simulink model "QiMotorController_ModelReference"  (R2021b)
settings: Solver=FixedStepDiscrete  StartTime=0.0  StopTime=5  RelTol=1e-3
PreLoadFcn:
  | RTWConfigurationCB('preloadfcn', bdroot);
PostLoadFcn:
  | load('configuration/data_struct.mat');
  | load('configuration/fluxMaps_propMotor.mat');
  | load('configuration/parameterInit_PROP.mat');
  | load('configuration/parameterInit_PUMP.mat');
  | load('configuration/parameterInit_PITCH.mat');
  | load('configuration/parameterInit_TILT.mat');
  | %load('configuration/base_workspace_signal_definition.mat');
  | %load('resolvedatastores_to_baseworkspace_for_faster_simulation.mat');
model workspace (MAT data in the model file):
  ADC_CALIBRATION_SAMPLES : Simulink.Parameter (value not decoded)
  DEFAULT_RESOLVER_CONTROL_WORD : Simulink.Parameter (value not decoded)
  PLL_FREQUENCY : Simulink.Parameter (value not decoded)
  SIMULATION_OPTIONS : Simulink.Parameter (value not decoded)
  TARGET_CODE_GEN : Simulink.Parameter (value not decoded)
  Ts = 2.5e-07
symbols that are objects in the model workspace (value not decoded): PLL_FREQUENCY, TARGET_CODE_GEN
undefined symbols (not defined in the file): DEADTIME_NS__PITCH, DEADTIME_NS__PROP, DEADTIME_NS__PUMP, DEADTIME_NS__TILT, fIa_, fIb_, fIc_, fIdc_, fMotorEncoderFloat_, fMotorSensorSpeed_, fUa_, fUb_, fUc_, fUdc_, inbtilt, mdl_pitch_uiAPUFlags, mdl_pitch_uiFlags, modelData, oMot_, oOut_, opInputResolverData_, oPitch, oState_, PLANT_SPEED_QUADRATIC_COEFF__PUMP, POLE_PAIRS_INIT__PITCH, POLE_PAIRS_INIT__PROP, POLE_PAIRS_INIT__PUMP, POLE_PAIRS_INIT__TILT, PWM_FREQ_KHZ__PITCH, PWM_FREQ_KHZ__PROP, PWM_FREQ_KHZ__PUMP, R_PHASE_INIT__PITCH, R_PHASE_INIT__PROP, R_PHASE_INIT__TILT, R_PHASE_INIT_PLANT__PUMP, uiControlReadback_, uiGateDriverStatus_
libraries: simulink x51, spsSeriesRLCBranchLib x25, spsMosfetLib x24, powerlib_extras x24, spsCurrentMeasurementLib x17, spsVoltageMeasurementLib x17, spsPermanentMagnetSynchronousMachineLib x3, spsDCVoltageSourceLib x2, motorModelLibrary x2, slpidlib x2, cstblocks x1, spspowerguiLib x1
(part 3 of 5)

== system QiMotorController_ModelReference/pitchMotor/PWM_pitch ==
  pitchMotor_PWMticks : Inport
  Bus Creator1 : BusCreator  Inputs=6
  Center-Aligned PWM 3-Phase   Modulator2 : Subsystem
  Demux3 : Demux  Outputs=6
  Demux4 : Demux  Outputs=3
  Logical Operator{7..12} (6 alike) : Logic  IconShape=distinctive  AllPortsSameDT=off  OutDataTypeStr=boolean
  On Delay{6..11} (6 alike) : powerlib_extras/Discrete  Control Blocks/Discrete On//Off Delay  type_delay=On delay  delay=DEADTIME_NS__PITCH*10^-9  ic=0  Ts=Ts
      settings: SourceProductBaseCode=PS
  pitchMotor_enable : Constant  OutDataTypeStr=boolean  SampleTime=-1
  pitchMotor_PWMgates : Outport
  wires:
  Demux3/4 -> Logical Operator11/1
  Demux3/2 -> Logical Operator9/1
  Demux3/5 -> Logical Operator7/1
  pitchMotor_PWMticks/1 -> Demux4/1
  Logical Operator12/1 -> On Delay11/1
  Logical Operator8/1 -> On Delay6/1
  Demux4/3 -> Center-Aligned PWM 3-Phase   Modulator2/3(C_ticks)
  pitchMotor_enable/1 -> Logical Operator12/2, Logical Operator7/2, Logical Operator11/2, Logical Operator10/2, Logical Operator9/2, Logical Operator8/2
  Center-Aligned PWM 3-Phase   Modulator2/1(PWM Gates) -> Demux3/1
  Logical Operator9/1 -> On Delay7/1
  On Delay9/1 -> Bus Creator1/4  "pitchGate_Bbottom"
  Demux4/2 -> Center-Aligned PWM 3-Phase   Modulator2/2(B_ticks)
  Logical Operator7/1 -> On Delay10/1
  Demux3/6 -> Logical Operator12/1
  Demux4/1 -> Center-Aligned PWM 3-Phase   Modulator2/1(A_ticks)
  Demux3/3 -> Logical Operator10/1
  On Delay8/1 -> Bus Creator1/3  "pitchGate_Btop"
  On Delay11/1 -> Bus Creator1/6  "pitchGate_Cbottom"
  On Delay7/1 -> Bus Creator1/2  "pitchGate_Abottom"
  On Delay6/1 -> Bus Creator1/1  "pitchGate_Atop"
  On Delay10/1 -> Bus Creator1/5  "pitchGate_Ctop"
  Logical Operator11/1 -> On Delay9/1
  Bus Creator1/1 -> pitchMotor_PWMgates/1
  Demux3/1 -> Logical Operator8/1
  Logical Operator10/1 -> On Delay8/1

== system QiMotorController_ModelReference/pitchMotor/Sense1 ==
  Current Measurement : spsCurrentMeasurementLib/Current Measurement  Tag=PoWeRsYsTeMmEaSuReMeNt  PhasorSimulation=off  OutputType=Complex  PSBequivalent=0
      settings: AttributesFormatString=\n
  Current Measurement1 : spsCurrentMeasurementLib/Current Measurement  Tag=PoWeRsYsTeMmEaSuReMeNt  PhasorSimulation=off  OutputType=Complex  PSBequivalent=0
      settings: AttributesFormatString=\n
  Current Measurement2 : spsCurrentMeasurementLib/Current Measurement  Tag=PoWeRsYsTeMmEaSuReMeNt  PhasorSimulation=off  OutputType=Complex  PSBequivalent=0
      settings: AttributesFormatString=\n
  Mux1 : Mux  Inputs=3
  Mux2 : Mux  Inputs=3
  Rate Transition : RateTransition  OutPortSampleTime=Ts
  Rate Transition1 : RateTransition  OutPortSampleTime=Ts
  Voltage Measurement : spsVoltageMeasurementLib/Voltage Measurement  PhasorSimulation=off  OutputType=Complex  PSBequivalent=0
  Voltage Measurement1 : spsVoltageMeasurementLib/Voltage Measurement  PhasorSimulation=off  OutputType=Complex  PSBequivalent=0
  Voltage Measurement2 : spsVoltageMeasurementLib/Voltage Measurement  PhasorSimulation=off  OutputType=Complex  PSBequivalent=0
  Ta : PMIOPort  Side=Left
  Tb : PMIOPort  Port=2  Side=Left
  Tc : PMIOPort  Port=3  Side=Left
  Mta : PMIOPort  Port=4  Side=Right
  Mtb : PMIOPort  Port=5  Side=Right
  Mtc : PMIOPort  Port=6  Side=Right
  Neutral : PMIOPort  Port=7  Side=Left
  I_abc : Outport  SampleTime=Ts
  V_abc : Outport  Port=2
  wires:
  Mux1/1 -> Rate Transition/1
  Current Measurement1/1 -> Mux1/2
  Current Measurement/1 -> Mux1/1
  Current Measurement2/1 -> Mux1/3
  Voltage Measurement/1 -> Mux2/1  "Van"
  Voltage Measurement1/1 -> Mux2/2  "Vbn"
  Voltage Measurement2/1 -> Mux2/3  "Vcn"
  Rate Transition/1 -> I_abc/1
  Mux2/1 -> Rate Transition1/1
  Rate Transition1/1 -> V_abc/1
  connections:
  Current Measurement2/RConn1 -- Mtc/RConn1
  Tc/RConn1 -- Voltage Measurement2/LConn1 -- Current Measurement2/LConn1
  Ta/RConn1 -- Voltage Measurement/LConn1 -- Current Measurement/LConn1
  Current Measurement/RConn1 -- Mta/RConn1
  Tb/RConn1 -- Voltage Measurement1/LConn1 -- Current Measurement1/LConn1
  Current Measurement1/RConn1 -- Mtb/RConn1
  Neutral/RConn1 -- Voltage Measurement1/LConn2 -- Voltage Measurement2/LConn2 -- Voltage Measurement/LConn2

== system QiMotorController_ModelReference/propMotor/PWM_prop ==
  propMotor_PWMticks : Inport
  Bus Creator : BusCreator  Inputs=6
  Center-Aligned PWM 3-Phase   Modulator1 : Subsystem
  Demux1 : Demux  Outputs=3
  Demux2 : Demux  Outputs=6
  Logical Operator{1..6} (6 alike) : Logic  IconShape=distinctive  AllPortsSameDT=off  OutDataTypeStr=boolean
  On Delay{,1..5} (6 alike) : powerlib_extras/Discrete  Control Blocks/Discrete On//Off Delay  type_delay=On delay  delay=DEADTIME_NS__PROP*10^-9  ic=0  Ts=Ts
      settings: SourceProductBaseCode=PS
  propMotor_enable : Constant  OutDataTypeStr=boolean  SampleTime=-1
  propMotor_PWMgates : Outport
  wires:
  Demux2/5 -> Logical Operator1/1
  Demux1/1 -> Center-Aligned PWM 3-Phase   Modulator1/1(Ua)
  Demux2/3 -> Logical Operator4/1
  Logical Operator3/1 -> On Delay1/1
  Demux2/1 -> Logical Operator2/1
  On Delay3/1 -> Bus Creator/4  "propGate_Bbottom"
  Logical Operator6/1 -> On Delay5/1
  Demux2/2 -> Logical Operator3/1
  Bus Creator/1 -> propMotor_PWMgates/1
  On Delay2/1 -> Bus Creator/3  "propGate_Btop"
  Demux1/3 -> Center-Aligned PWM 3-Phase   Modulator1/3(Uc)
  On Delay1/1 -> Bus Creator/2  "propGate_Abottom"
  Center-Aligned PWM 3-Phase   Modulator1/1(PWM Gates) -> Demux2/1
  Demux2/4 -> Logical Operator5/1
  Logical Operator5/1 -> On Delay3/1
  propMotor_enable/1 -> Logical Operator6/2, Logical Operator1/2, Logical Operator5/2, Logical Operator4/2, Logical Operator3/2, Logical Operator2/2
  Demux1/2 -> Center-Aligned PWM 3-Phase   Modulator1/2(Ub)
  On Delay/1 -> Bus Creator/1  "propGate_Atop"
  On Delay5/1 -> Bus Creator/6  "propGate_Cbottom"
  Logical Operator4/1 -> On Delay2/1
  propMotor_PWMticks/1 -> Demux1/1
  Demux2/6 -> Logical Operator6/1
  On Delay4/1 -> Bus Creator/5  "propGate_Ctop"
  Logical Operator2/1 -> On Delay/1
  Logical Operator1/1 -> On Delay4/1

== system QiMotorController_ModelReference/propMotor/Sense1 ==
  Current Measurement : spsCurrentMeasurementLib/Current Measurement  Tag=PoWeRsYsTeMmEaSuReMeNt  PhasorSimulation=off  OutputType=Complex  PSBequivalent=0
      settings: AttributesFormatString=\n
  Current Measurement1 : spsCurrentMeasurementLib/Current Measurement  Tag=PoWeRsYsTeMmEaSuReMeNt  PhasorSimulation=off  OutputType=Complex  PSBequivalent=0
      settings: AttributesFormatString=\n
  Current Measurement2 : spsCurrentMeasurementLib/Current Measurement  Tag=PoWeRsYsTeMmEaSuReMeNt  PhasorSimulation=off  OutputType=Complex  PSBequivalent=0
      settings: AttributesFormatString=\n
  Mux1 : Mux  Inputs=3
  Mux2 : Mux  Inputs=3
  Rate Transition : RateTransition  OutPortSampleTime=Ts
  Rate Transition1 : RateTransition  OutPortSampleTime=Ts
  Voltage Measurement : spsVoltageMeasurementLib/Voltage Measurement  PhasorSimulation=off  OutputType=Complex  PSBequivalent=0
  Voltage Measurement1 : spsVoltageMeasurementLib/Voltage Measurement  PhasorSimulation=off  OutputType=Complex  PSBequivalent=0
  Voltage Measurement2 : spsVoltageMeasurementLib/Voltage Measurement  PhasorSimulation=off  OutputType=Complex  PSBequivalent=0
  Ta : PMIOPort  Side=Left
  Tb : PMIOPort  Port=2  Side=Left
  Tc : PMIOPort  Port=3  Side=Left
  Mta : PMIOPort  Port=4  Side=Right
  Mtb : PMIOPort  Port=5  Side=Right
  Mtc : PMIOPort  Port=6  Side=Right
  Neutral : PMIOPort  Port=7  Side=Left
  I_abc : Outport  SampleTime=Ts
  V_abc : Outport  Port=2
  wires:
  Mux1/1 -> Rate Transition/1
  Current Measurement1/1 -> Mux1/2
  Current Measurement/1 -> Mux1/1
  Current Measurement2/1 -> Mux1/3
  Voltage Measurement/1 -> Mux2/1  "Van"
  Voltage Measurement1/1 -> Mux2/2  "Vbn"
  Voltage Measurement2/1 -> Mux2/3  "Vcn"
  Rate Transition/1 -> I_abc/1
  Mux2/1 -> Rate Transition1/1
  Rate Transition1/1 -> V_abc/1
  connections:
  Current Measurement2/RConn1 -- Mtc/RConn1
  Tc/RConn1 -- Voltage Measurement2/LConn1 -- Current Measurement2/LConn1
  Ta/RConn1 -- Voltage Measurement/LConn1 -- Current Measurement/LConn1
  Current Measurement/RConn1 -- Mta/RConn1
  Tb/RConn1 -- Voltage Measurement1/LConn1 -- Current Measurement1/LConn1
  Current Measurement1/RConn1 -- Mtb/RConn1
  Neutral/RConn1 -- Voltage Measurement1/LConn2 -- Voltage Measurement2/LConn2 -- Voltage Measurement/LConn2

== system QiMotorController_ModelReference/propMotor/Sim Option Prop Variant Subsystem ==
  note: 1) Add Subsystem or Model blocks as valid variant choices.
      | 2) You cannot connect blocks at this level. At simulation, connectivity is automatically
      | determined, based on the active variant and port name matching.
  In1 : Inport
  Sim Options 0 Prop Subsystem : Subsystem  VariantControl=(default)
  Sim Options 1 Prop Subsystem : Subsystem  VariantControl=SIMULATION_OPTIONS == 1 && TARGET_CODE_GEN ~= 1
  Out1 : Outport

== system QiMotorController_ModelReference/pumpfanMotor/PWM_pumpfan ==
  pumpMotor_PWMticks : Inport
  Bus Creator : BusCreator  Inputs=6
  Center-Aligned PWM 3-Phase   Modulator1 : Subsystem
  Demux1 : Demux  Outputs=3
  Demux2 : Demux  Outputs=6
  Logical Operator{1..6} (6 alike) : Logic  IconShape=distinctive  AllPortsSameDT=off  OutDataTypeStr=boolean
  On Delay{,1..5} (6 alike) : powerlib_extras/Discrete  Control Blocks/Discrete On//Off Delay  type_delay=On delay  delay=DEADTIME_NS__PUMP*10^-9  ic=0  Ts=Ts
      settings: SourceProductBaseCode=PS
  pumpMotor_enable : Constant  OutDataTypeStr=boolean  SampleTime=-1
  pumpMotor_PWMgates : Outport
  wires:
  Demux2/5 -> Logical Operator1/1
  Demux1/1 -> Center-Aligned PWM 3-Phase   Modulator1/1(Ua)
  Demux2/3 -> Logical Operator4/1
  Logical Operator3/1 -> On Delay1/1
  Demux2/1 -> Logical Operator2/1
  On Delay3/1 -> Bus Creator/4  "pumpGate_Bbottom"
  Logical Operator6/1 -> On Delay5/1
  Demux2/2 -> Logical Operator3/1
  Bus Creator/1 -> pumpMotor_PWMgates/1
  On Delay2/1 -> Bus Creator/3  "pumpGate_Btop"
  Demux1/3 -> Center-Aligned PWM 3-Phase   Modulator1/3(Uc)
  On Delay1/1 -> Bus Creator/2  "pumpGate_Abottom"
  Center-Aligned PWM 3-Phase   Modulator1/1(PWM Gates) -> Demux2/1
  Demux2/4 -> Logical Operator5/1
  Logical Operator5/1 -> On Delay3/1
  pumpMotor_enable/1 -> Logical Operator6/2, Logical Operator1/2, Logical Operator5/2, Logical Operator4/2, Logical Operator3/2, Logical Operator2/2
  Demux1/2 -> Center-Aligned PWM 3-Phase   Modulator1/2(Ub)
  On Delay/1 -> Bus Creator/1  "pumpGate_Atop"
  On Delay5/1 -> Bus Creator/6  "pumpGate_Cbottom"
  Logical Operator4/1 -> On Delay2/1
  pumpMotor_PWMticks/1 -> Demux1/1
  Demux2/6 -> Logical Operator6/1
  On Delay4/1 -> Bus Creator/5  "pumpGate_Ctop"
  Logical Operator2/1 -> On Delay/1
  Logical Operator1/1 -> On Delay4/1

== system QiMotorController_ModelReference/pumpfanMotor/Sense1 ==
  Current Measurement : spsCurrentMeasurementLib/Current Measurement  Tag=PoWeRsYsTeMmEaSuReMeNt  PhasorSimulation=off  OutputType=Complex  PSBequivalent=0
      settings: AttributesFormatString=\n
  Current Measurement1 : spsCurrentMeasurementLib/Current Measurement  Tag=PoWeRsYsTeMmEaSuReMeNt  PhasorSimulation=off  OutputType=Complex  PSBequivalent=0
      settings: AttributesFormatString=\n
  Current Measurement2 : spsCurrentMeasurementLib/Current Measurement  Tag=PoWeRsYsTeMmEaSuReMeNt  PhasorSimulation=off  OutputType=Complex  PSBequivalent=0
      settings: AttributesFormatString=\n
  Mux1 : Mux  Inputs=3
  Mux2 : Mux  Inputs=3
  Rate Transition : RateTransition  OutPortSampleTime=Ts
  Rate Transition1 : RateTransition  OutPortSampleTime=Ts
  Voltage Measurement : spsVoltageMeasurementLib/Voltage Measurement  PhasorSimulation=off  OutputType=Complex  PSBequivalent=0
  Voltage Measurement1 : spsVoltageMeasurementLib/Voltage Measurement  PhasorSimulation=off  OutputType=Complex  PSBequivalent=0
  Voltage Measurement2 : spsVoltageMeasurementLib/Voltage Measurement  PhasorSimulation=off  OutputType=Complex  PSBequivalent=0
  Ta : PMIOPort  Side=Left
  Tb : PMIOPort  Port=2  Side=Left
  Tc : PMIOPort  Port=3  Side=Left
  Mta : PMIOPort  Port=4  Side=Right
  Mtb : PMIOPort  Port=5  Side=Right
  Mtc : PMIOPort  Port=6  Side=Right
  Neutral : PMIOPort  Port=7  Side=Left
  I_abc : Outport  SampleTime=Ts
  V_abc : Outport  Port=2
  wires:
  Mux1/1 -> Rate Transition/1
  Current Measurement1/1 -> Mux1/2
  Current Measurement/1 -> Mux1/1
  Current Measurement2/1 -> Mux1/3
  Voltage Measurement/1 -> Mux2/1  "Van"
  Voltage Measurement1/1 -> Mux2/2  "Vbn"
  Voltage Measurement2/1 -> Mux2/3  "Vcn"
  Rate Transition/1 -> I_abc/1
  Mux2/1 -> Rate Transition1/1
  Rate Transition1/1 -> V_abc/1
  connections:
  Current Measurement2/RConn1 -- Mtc/RConn1
  Tc/RConn1 -- Voltage Measurement2/LConn1 -- Current Measurement2/LConn1
  Ta/RConn1 -- Voltage Measurement/LConn1 -- Current Measurement/LConn1
  Current Measurement/RConn1 -- Mta/RConn1
  Tb/RConn1 -- Voltage Measurement1/LConn1 -- Current Measurement1/LConn1
  Current Measurement1/RConn1 -- Mtb/RConn1
  Neutral/RConn1 -- Voltage Measurement1/LConn2 -- Voltage Measurement2/LConn2 -- Voltage Measurement/LConn2

== system QiMotorController_ModelReference/pumpfanMotor/Sim Option Pump Variant Subsystem ==
  note: 1) Add Subsystem or Model blocks as valid variant choices.
      | 2) You cannot connect blocks at this level. At simulation, connectivity is automatically
      | determined, based on the active variant and port name matching.
  In1 : Inport
  Sim Options 0 Pump Subsystem : Subsystem  VariantControl=(default)
  Sim Options 1 Pump Subsystem : Subsystem  VariantControl=SIMULATION_OPTIONS == 1 && TARGET_CODE_GEN ~= 1
  Out1 : Outport

== system QiMotorController_ModelReference/tiltMotor/PWM_tilt ==
  tiltMotor_PWMticks : Inport
  Bus Creator1 : BusCreator  Inputs=6
  Center-Aligned PWM 3-Phase   Modulator2 : Subsystem
  Demux3 : Demux  Outputs=6
  Demux4 : Demux  Outputs=3
  Logical Operator{7..12} (6 alike) : Logic  IconShape=distinctive  AllPortsSameDT=off  OutDataTypeStr=boolean
  On Delay{6..11} (6 alike) : powerlib_extras/Discrete  Control Blocks/Discrete On//Off Delay  type_delay=On delay  delay=DEADTIME_NS__TILT*10^-9  ic=0  Ts=Ts
      settings: SourceProductBaseCode=PS
  tiltMotor_enable : Constant  OutDataTypeStr=boolean  SampleTime=-1
  tiltMotor_PWMgates : Outport
  wires:
  Demux3/4 -> Logical Operator11/1
  Demux3/2 -> Logical Operator9/1
  Demux3/5 -> Logical Operator7/1
  tiltMotor_PWMticks/1 -> Demux4/1
  Logical Operator12/1 -> On Delay11/1
  Logical Operator8/1 -> On Delay6/1
  Demux4/3 -> Center-Aligned PWM 3-Phase   Modulator2/3(C_ticks)
  tiltMotor_enable/1 -> Logical Operator12/2, Logical Operator7/2, Logical Operator11/2, Logical Operator10/2, Logical Operator9/2, Logical Operator8/2
  Center-Aligned PWM 3-Phase   Modulator2/1(PWM Gates) -> Demux3/1
  Logical Operator9/1 -> On Delay7/1
  On Delay9/1 -> Bus Creator1/4  "tiltGate_Bbottom"
  Demux4/2 -> Center-Aligned PWM 3-Phase   Modulator2/2(B_ticks)
  Logical Operator7/1 -> On Delay10/1
  Demux3/6 -> Logical Operator12/1
  Demux4/1 -> Center-Aligned PWM 3-Phase   Modulator2/1(A_ticks)
  Demux3/3 -> Logical Operator10/1
  On Delay8/1 -> Bus Creator1/3  "tiltGate_Btop"
  On Delay11/1 -> Bus Creator1/6  "tiltGate_Cbottom"
  On Delay7/1 -> Bus Creator1/2  "tiltGate_Abottom"
  On Delay6/1 -> Bus Creator1/1  "tiltGate_Atop"
  On Delay10/1 -> Bus Creator1/5  "tiltGate_Ctop"
  Logical Operator11/1 -> On Delay9/1
  Bus Creator1/1 -> tiltMotor_PWMgates/1
  Demux3/1 -> Logical Operator8/1
  Logical Operator10/1 -> On Delay8/1

== system QiMotorController_ModelReference/tiltMotor/Sense1 ==
  Current Measurement : spsCurrentMeasurementLib/Current Measurement  Tag=PoWeRsYsTeMmEaSuReMeNt  PhasorSimulation=off  OutputType=Complex  PSBequivalent=0
      settings: AttributesFormatString=\n
  Current Measurement1 : spsCurrentMeasurementLib/Current Measurement  Tag=PoWeRsYsTeMmEaSuReMeNt  PhasorSimulation=off  OutputType=Complex  PSBequivalent=0
      settings: AttributesFormatString=\n
  Current Measurement2 : spsCurrentMeasurementLib/Current Measurement  Tag=PoWeRsYsTeMmEaSuReMeNt  PhasorSimulation=off  OutputType=Complex  PSBequivalent=0
      settings: AttributesFormatString=\n
  Mux1 : Mux  Inputs=3
  Mux2 : Mux  Inputs=3
  Rate Transition : RateTransition  OutPortSampleTime=Ts
  Rate Transition1 : RateTransition  OutPortSampleTime=Ts
  Voltage Measurement : spsVoltageMeasurementLib/Voltage Measurement  PhasorSimulation=off  OutputType=Complex  PSBequivalent=0
  Voltage Measurement1 : spsVoltageMeasurementLib/Voltage Measurement  PhasorSimulation=off  OutputType=Complex  PSBequivalent=0
  Voltage Measurement2 : spsVoltageMeasurementLib/Voltage Measurement  PhasorSimulation=off  OutputType=Complex  PSBequivalent=0
  Ta : PMIOPort  Side=Left
  Tb : PMIOPort  Port=2  Side=Left
  Tc : PMIOPort  Port=3  Side=Left
  Mta : PMIOPort  Port=4  Side=Right
  Mtb : PMIOPort  Port=5  Side=Right
  Mtc : PMIOPort  Port=6  Side=Right
  Neutral : PMIOPort  Port=7  Side=Left
  I_abc : Outport  SampleTime=Ts
  V_abc : Outport  Port=2
  wires:
  Mux1/1 -> Rate Transition/1
  Current Measurement1/1 -> Mux1/2
  Current Measurement/1 -> Mux1/1
  Current Measurement2/1 -> Mux1/3
  Voltage Measurement/1 -> Mux2/1  "Van"
  Voltage Measurement1/1 -> Mux2/2  "Vbn"
  Voltage Measurement2/1 -> Mux2/3  "Vcn"
  Rate Transition/1 -> I_abc/1
  Mux2/1 -> Rate Transition1/1
  Rate Transition1/1 -> V_abc/1
  connections:
  Current Measurement2/RConn1 -- Mtc/RConn1
  Tc/RConn1 -- Voltage Measurement2/LConn1 -- Current Measurement2/LConn1
  Ta/RConn1 -- Voltage Measurement/LConn1 -- Current Measurement/LConn1
  Current Measurement/RConn1 -- Mta/RConn1
  Tb/RConn1 -- Voltage Measurement1/LConn1 -- Current Measurement1/LConn1
  Current Measurement1/RConn1 -- Mtb/RConn1
  Neutral/RConn1 -- Voltage Measurement1/LConn2 -- Voltage Measurement2/LConn2 -- Voltage Measurement/LConn2

== system QiMotorController_ModelReference/Fault Injection/pitchMotor_faults/DC Current Disturbance ==
  Idc_feedback : Inport
  Idc_value : Inport  Port=2
  Abs1 : Abs
  Constant2 : Constant  Value=0  OutDataTypeStr=single  SampleTime=-1
  GreaterThan1 : RelationalOperator  Operator=>  OutDataTypeStr=boolean  RndMeth=Simplest
  Switch : Switch  Criteria=u2 > Threshold
  Idc_fault : Outport
  wires:
  Idc_feedback/1 -> Switch/3
  GreaterThan1/1 -> Switch/2
  Switch/1 -> Idc_fault/1
  Idc_value/1 -> Switch/1, Abs1/1
  Constant2/1 -> GreaterThan1/2
  Abs1/1 -> GreaterThan1/1

== system QiMotorController_ModelReference/Fault Injection/pitchMotor_faults/DC Voltage Disturbance ==
  Udc_feedback : Inport
  Udc_value : Inport  Port=2
  Constant1 : Constant  Value=0  OutDataTypeStr=single  SampleTime=-1
  GreaterThan : RelationalOperator  Operator=>  OutDataTypeStr=boolean  RndMeth=Simplest
  Switch : Switch  Criteria=u2 > Threshold
  Udc_fault : Outport
  wires:
  Udc_value/1 -> Switch/1, GreaterThan/1
  GreaterThan/1 -> Switch/2
  Constant1/1 -> GreaterThan/2
  Udc_feedback/1 -> Switch/3
  Switch/1 -> Udc_fault/1

== system QiMotorController_ModelReference/Fault Injection/pitchMotor_faults/Phase Current & Aux Disturbances ==
  note: This simulates a HW overcurrent fault (1008) coming from the FPGA.
      | Takes precedence over other faults.
  Iabc_feedback : Inport
  IphMagnitude_value : Inport  Port=2
  Target_phase : Inport  Port=3
  Aux_trip_code : Inport  Port=4
  uiGateDriverStatus : Inport  Port=5
  mdl_pitch_uiFlags : Inport  Port=6
  mdl_pitch_uiAPUFlags : Inport  Port=7
  Constant : Constant  Value=0xF  OutDataTypeStr=uint32  SampleTime=-1
  Constant2 : Constant  Value=10  OutDataTypeStr=single  SampleTime=-1
  Fault Current Setting : Subsystem
  GreaterThan1 : RelationalOperator  Operator=>  OutDataTypeStr=boolean  RndMeth=Simplest
  Set uiAPUFlags for Aux Trips : Subsystem  TreatAsAtomicUnit=on
  Set uiFlags for Aux Trips : Subsystem  TreatAsAtomicUnit=on
  Set uiGateDriverStatus for Aux Trips : Subsystem  TreatAsAtomicUnit=on
  Switch1 : Switch  Criteria=u2 > Threshold
  Iabc_fault : Outport
  uiGateDriverStatus_fault : Outport  Port=2
  uiFlags_fault : Outport  Port=3
  uiAPUFlags_fault : Outport  Port=4
  wires:
  IphMagnitude_value/1 -> Fault Current Setting/3(IphMagnitude_value), GreaterThan1/1
  Constant2/1 -> GreaterThan1/2
  GreaterThan1/1 -> Switch1/2
  Switch1/1 -> uiGateDriverStatus_fault/1
  Constant/1 -> Switch1/1
  Target_phase/1 -> Fault Current Setting/1(targetPhase)
  Aux_trip_code/1 -> Set uiAPUFlags for Aux Trips/1(auxTripCode), Set uiFlags for Aux Trips/1(auxTripCode), Set uiGateDriverStatus for Aux Trips/1(auxTripCode)
  mdl_pitch_uiFlags/1 -> Set uiFlags for Aux Trips/2(uiFlags)
  uiGateDriverStatus/1 -> Set uiGateDriverStatus for Aux Trips/2(uiGateDriverStatus)
  Set uiGateDriverStatus for Aux Trips/1(uiGateDriverStatus_fault) -> Switch1/3
  Set uiFlags for Aux Trips/1(uiFlags_fault) -> uiFlags_fault/1
  Iabc_feedback/1 -> Fault Current Setting/2(Iabc_feedback)
  Fault Current Setting/1(Iabc_fault) -> Iabc_fault/1
  Set uiAPUFlags for Aux Trips/1(uiAPUFlags_fault) -> uiAPUFlags_fault/1
  mdl_pitch_uiAPUFlags/1 -> Set uiAPUFlags for Aux Trips/2(uiAPUFlags)

== system QiMotorController_ModelReference/Fault Injection/pitchMotor_faults/Position Control Disturbances ==
  uiControlFeedback : Inport
  uiControlFeedback_value : Inport  Port=2
  Constant1 : Constant  Value=0  OutDataTypeStr=uint32  SampleTime=-1
  Constant2 : Constant  Value=0  OutDataTypeStr=uint32  SampleTime=-1
  GreaterThan1 : RelationalOperator  Operator=>  OutDataTypeStr=boolean  RndMeth=Simplest
  Switch : Switch  Criteria=u2 > Threshold
  uiControlFeedback_fault : Outport
  wires:
  uiControlFeedback/1 -> Switch/3
  GreaterThan1/1 -> Switch/2
  Switch/1 -> uiControlFeedback_fault/1
  uiControlFeedback_value/1 -> GreaterThan1/1
  Constant2/1 -> GreaterThan1/2
  Constant1/1 -> Switch/1

== system QiMotorController_ModelReference/InboardTiltDragLaw2/drag2/coulomb_drag_logic ==
  Bus Element In2 : Inport  PortName=velocity_m
  Bus Element In : Inport  Port=2  PortName=net_torque_m
  Bus Element In3 : Inport  Port=2  PortName=net_torque_m
  Bus Element In1 : Inport  Port=3  PortName=nominal_drag_torque_m
  Bus Element In4 : Inport  Port=3  PortName=nominal_drag_torque_m
  AND : Logic  IconShape=distinctive  AllPortsSameDT=off  OutDataTypeStr=boolean
  Abs5 : Abs
  Equal : RelationalOperator  Operator=<  OutDataTypeStr=boolean  RndMeth=Simplest
  Less Than : RelationalOperator  Operator=<  OutDataTypeStr=boolean  RndMeth=Simplest
  Product1 : Product
  Sign1 : Signum
  Switch : Switch  Criteria=u2 > Threshold
  minimum_stick_slip_velocity : Constant  Value=2e-1  OutDataTypeStr=Inherit: Inherit via back propagation
  Bus Element Out : Outport  PortName=drag_torque_out_m
  wires:
  Product1/1 -> Bus Element Out/1  "drag"
  Switch/1 -> Product1/2
  Sign1/1 -> Product1/1  "sgn"
  Bus Element In4/1 -> Switch/3
  Bus Element In1/1 -> Less Than/2  "nomtq"
  Bus Element In3/1 -> Switch/1  "nettq"
  Less Than/1 -> AND/2
  AND/1 -> Switch/2  "drag_conditional"
  Bus Element In2/1 -> Abs5/1, Sign1/1  "vm"
  Abs5/1 -> Equal/1
  Equal/1 -> AND/1
  minimum_stick_slip_velocity/1 -> Equal/2
  Bus Element In/1 -> Less Than/1  "nettq"

== system QiMotorController_ModelReference/InboardTiltDragLaw2/drag2/load ==
  Bus Element In4 : Inport  PortName=velocity_m
  Bus Element In1 : Inport  Port=2  PortName=ideal_load_torque_m
  Bus Element In2 : Inport  Port=2  PortName=ideal_load_torque_m
  Bus Element In3 : Inport  Port=2  PortName=ideal_load_torque_m
  Bus Element In14 : Inport  Port=3  PortName=motor_temp
  Bus Element In5 : Inport  Port=4  PortName=n_invs
  Abs2 : Abs
  Display : Display
  Display1 : Display
  Product : Product
  Product2 : Product
  Switch : Switch  Criteria=u2 > Threshold
  direct_efficiency : Subsystem
  e1 : Lookup_n-D  BreakpointsForDimension1=inbtilt.EfficiencyTemperatureBreakpoints  BreakpointsForDimension2=inbtilt.EfficiencySpeedBreakpoints  Table=inbtilt.EfficiencyTable  InternalRulePriority=Speed  RndMeth=Simplest  InputSameDT=on
      settings: InputPortMap=u0,u1
  indirect_efficiency_reduction : Subsystem
  Bus Element Out1 : Outport  PortName=load_torque
  wires:
  e1/1 -> direct_efficiency/1(table_efficiency)
  Bus Element In3/1 -> direct_efficiency/3(ideal_load_torque_m)
  Bus Element In2/1 -> Product2/2, Display/1
  Product2/1 -> Bus Element Out1/1
  Bus Element In1/1 -> indirect_efficiency_reduction/1(torque_load_m)
  indirect_efficiency_reduction/1(efficiency_load_reduction) -> Product/2
  Product/1 -> Switch/3  "e_indirect"
  Bus Element In5/1 -> Switch/2
  Switch/1 -> Product2/1, Display1/1  "e"
  direct_efficiency/1(nominal_efficiency) -> Switch/1, Product/1  "e_direct"
  Abs2/1 -> e1/2  "vm"
  Bus Element In14/1 -> e1/1  "T"
  Bus Element In4/1 -> direct_efficiency/2(velocity_m), Abs2/1

== system QiMotorController_ModelReference/Signal Conditioning/qi_dsm_to_sinc1/compute_dsm_output ==
  sig_in : Inport
  Add : Sum  Inputs=+-
  Add{1,3..7} (6 alike) : Sum
  Add2 : Sum  Inputs=+-
  Compare To Constant : simulink/Logic and Bit Operations/Compare To Constant  relop=>=  const=0  OutDataTypeStr=boolean
  Constant : Constant  SampleTime=-1
  Constant1 : Constant  Value=0  SampleTime=-1
  Constant2 : Constant  SampleTime=-1
  Constant3 : Constant  Value=2  SampleTime=-1
  Divide{,1..7} (8 alike) : Product  Inputs=**
  Switch : Switch  Criteria=u2 > Threshold
  Switch1 : Switch  Criteria=u2 > Threshold
  Switch2 : Switch  Criteria=u2 > Threshold
  Unit Delay{,1..6} (7 alike) : UnitDelay  SampleTime=-1  HasFrameUpgradeWarning=on
  pdm_signal : Outport
  wires:
  [b2] -> Divide/1
  [vref] -> Divide/2
  [s1_accum] -> Unit Delay1/1
  Divide/1 -> Add/2
  [s2_accum] -> Unit Delay/1
  [a2] -> Divide1/1
  Add/1 -> Divide1/2
  Unit Delay1/1 -> Add/1
  Unit Delay/1 -> Add1/1
  Divide1/1 -> Add1/2
  [vref] -> Divide2/2
  [b1] -> Divide2/1
  Divide2/1 -> Add2/2
  [a1] -> Divide3/1
  Add2/1 -> Divide3/2
  [s1_accum] -> Unit Delay2/1
  Unit Delay2/1 -> Add3/1
  Divide3/1 -> Add3/2
  [s2_accum] -> Unit Delay3/1
  Unit Delay3/1 -> Compare To Constant/1
  Add1/1 -> Switch/1
  Add3/1 -> Switch1/1
  Switch1/1 -> [s1_accum]
  Switch/1 -> [s2_accum]
  Compare To Constant/1 -> Switch1/2, Switch/2, Switch2/2
  Switch2/1 -> [dout], pdm_signal/1
  Constant/1 -> Switch2/1
  Constant1/1 -> Switch2/3
  [s2_accum] -> Unit Delay4/1
  Unit Delay4/1 -> Add5/1
  [s1_accum] -> Unit Delay5/1
  [a2] -> Divide5/1
  [vref] -> Divide4/2
  Add4/1 -> Divide5/2
  Unit Delay5/1 -> Add4/1
  [b2] -> Divide4/1
  Add5/1 -> Switch/3
  Divide5/1 -> Add5/2
  Divide4/1 -> Add4/2
  [s1_accum] -> Unit Delay6/1
  [b1] -> Divide6/1
  Divide7/1 -> Add7/2
  Add7/1 -> Switch1/3
  [a1] -> Divide7/1
  sig_in/1 -> Add6/1, Add2/1
  Add6/1 -> Divide7/2
  Unit Delay6/1 -> Add7/1
  [vref] -> Divide6/2
  Divide6/1 -> Add6/2
  Constant2/1 -> [a2], [vref], [b1], [a1]
  Constant3/1 -> [b2]

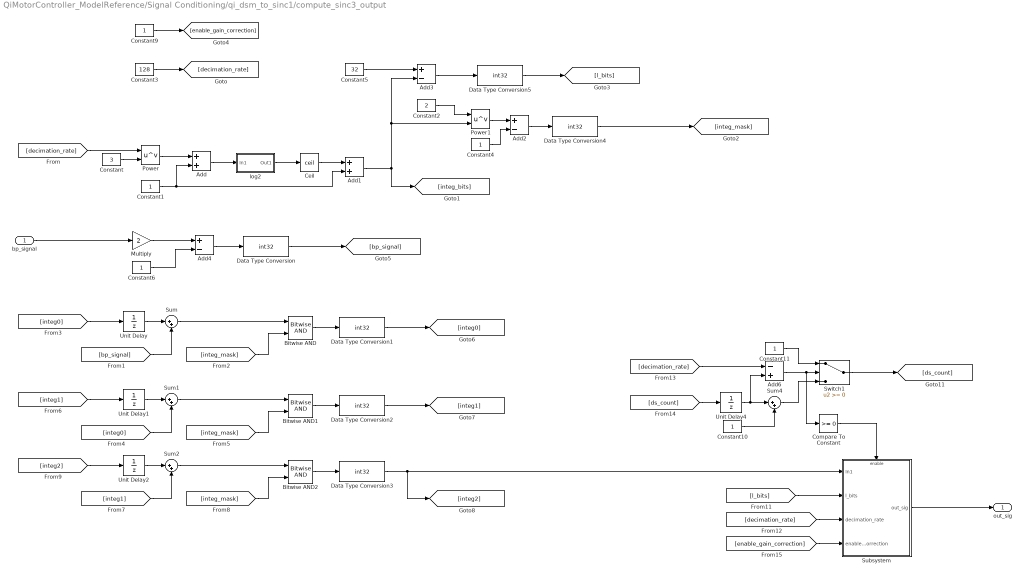
== system QiMotorController_ModelReference/Signal Conditioning/qi_dsm_to_sinc1/compute_sinc3_output ==
  bp_signal : Inport
  Add : Sum
  Add1 : Sum
  Add2 : Sum  Inputs=+-
  Add3 : Sum  Inputs=+-
  Add4 : Sum  Inputs=+-  OutDataTypeStr=int32
  Add6 : Sum  Inputs=-+  OutDataTypeStr=int32
  Bitwise AND : simulink/Logic and Bit Operations/Bitwise Operator  logicop=AND  UseBitMask=off  NumInputPorts=2  BitMask=bin2dec('11011001')  BitMaskRealWorld=Stored Integer
  Bitwise AND1 : simulink/Logic and Bit Operations/Bitwise Operator  logicop=AND  UseBitMask=off  NumInputPorts=2  BitMask=bin2dec('11011001')  BitMaskRealWorld=Stored Integer
  Bitwise AND2 : simulink/Logic and Bit Operations/Bitwise Operator  logicop=AND  UseBitMask=off  NumInputPorts=2  BitMask=bin2dec('11011001')  BitMaskRealWorld=Stored Integer
  Ceil : Rounding  Operator=ceil
  Compare To Constant : simulink/Logic and Bit Operations/Compare To Constant  relop=>=  const=0  OutDataTypeStr=boolean
  Constant : Constant  Value=3  OutDataTypeStr=single  SampleTime=-1
  Constant1 : Constant  OutDataTypeStr=single  SampleTime=-1
  Constant10 : Constant  OutDataTypeStr=int32  SampleTime=-1
  Constant11 : Constant  OutDataTypeStr=int32  SampleTime=-1
  Constant2 : Constant  Value=2  OutDataTypeStr=single  SampleTime=-1
  Constant3 : Constant  Value=128  OutDataTypeStr=single  SampleTime=-1
  Constant4 : Constant  OutDataTypeStr=single  SampleTime=-1
  Constant5 : Constant  Value=32  OutDataTypeStr=single  SampleTime=-1
  Constant6 : Constant  OutDataTypeStr=single  SampleTime=-1
  Constant9 : Constant  OutDataTypeStr=boolean  SampleTime=-1
  Data Type Conversion{,1..5} (6 alike) : DataTypeConversion  OutDataTypeStr=int32
  Multiply : Gain  Gain=2
  Power : Math  Operator=pow  SaturateOnIntegerOverflow=on
  Power1 : Math  Operator=pow  SaturateOnIntegerOverflow=on
  Subsystem : Subsystem
  Sum{,1..2,4} (4 alike) : Sum  Inputs=|++
  Switch1 : Switch
  Unit Delay : UnitDelay  SampleTime=-1  HasFrameUpgradeWarning=on
  Unit Delay1 : UnitDelay  SampleTime=-1  HasFrameUpgradeWarning=on
  Unit Delay2 : UnitDelay  SampleTime=-1  HasFrameUpgradeWarning=on
  Unit Delay4 : UnitDelay  InitialCondition=1  SampleTime=-1  HasFrameUpgradeWarning=on
  log2 : Subsystem
  out_sig : Outport
  wires:
  [decimation_rate] -> Power/1
  Constant/1 -> Power/2
  Power/1 -> Add/1
  Constant1/1 -> Add1/2, Add/2
  Constant3/1 -> [decimation_rate]
  Add/1 -> log2/1(In1)
  log2/1(Out1) -> Ceil/1
  Ceil/1 -> Add1/1
  Add1/1 -> Add3/2, Power1/2, [integ_bits]
  Constant2/1 -> Power1/1
  Power1/1 -> Add2/1
  Constant4/1 -> Add2/2
  Add2/1 -> Data Type Conversion4/1
  Constant5/1 -> Add3/1
  Add3/1 -> Data Type Conversion5/1
  bp_signal/1 -> Multiply/1
  Multiply/1 -> Add4/1
  Constant6/1 -> Add4/2
  Add4/1 -> Data Type Conversion/1
  Data Type Conversion/1 -> [bp_signal]
  Sum/1 -> Bitwise AND/1
  Unit Delay/1 -> Sum/1
  [bp_signal] -> Sum/2
  [integ_mask] -> Bitwise AND/2
  Bitwise AND/1 -> Data Type Conversion1/1
  Data Type Conversion1/1 -> [integ0]
  [integ0] -> Unit Delay/1
  Bitwise AND1/1 -> Data Type Conversion2/1
  [integ1] -> Unit Delay1/1
  [integ_mask] -> Bitwise AND1/2
  Unit Delay1/1 -> Sum1/1
  Sum1/1 -> Bitwise AND1/1
  [integ0] -> Sum1/2
  Unit Delay2/1 -> Sum2/1
  Bitwise AND2/1 -> Data Type Conversion3/1
  [integ1] -> Sum2/2
  [integ2] -> Unit Delay2/1
  Sum2/1 -> Bitwise AND2/1
  [integ_mask] -> Bitwise AND2/2
  Data Type Conversion4/1 -> [integ_mask]
  Data Type Conversion5/1 -> [l_bits]
  Constant9/1 -> [enable_gain_correction]
  Subsystem/1(out_sig) -> out_sig/1
  Sum4/1 -> Switch1/3
  Constant10/1 -> Sum4/2
  Unit Delay4/1 -> Sum4/1, Add6/2
  Constant11/1 -> Switch1/1
  Switch1/1 -> [ds_count]
  [ds_count] -> Unit Delay4/1
  [decimation_rate] -> Add6/1
  Add6/1 -> Compare To Constant/1, Switch1/2
  Compare To Constant/1 -> Subsystem/Enable
  Data Type Conversion3/1 -> [integ2], Subsystem/1(In1)
  Data Type Conversion2/1 -> [integ1]
  [l_bits] -> Subsystem/2(l_bits)
  [decimation_rate] -> Subsystem/3(decimation_rate)
  [enable_gain_correction] -> Subsystem/4(enable_gain_correction)

== system QiMotorController_ModelReference/Signal Conditioning/qi_dsm_to_sinc2/compute_dsm_output ==
  sig_in : Inport
  Add : Sum  Inputs=+-
  Add{1,3..7} (6 alike) : Sum
  Add2 : Sum  Inputs=+-
  Compare To Constant : simulink/Logic and Bit Operations/Compare To Constant  relop=>=  const=0  OutDataTypeStr=boolean
  Constant : Constant  SampleTime=-1
  Constant1 : Constant  Value=0  SampleTime=-1
  Constant2 : Constant  SampleTime=-1
  Constant3 : Constant  Value=2  SampleTime=-1
  Divide{,1..7} (8 alike) : Product  Inputs=**
  Switch : Switch  Criteria=u2 > Threshold
  Switch1 : Switch  Criteria=u2 > Threshold
  Switch2 : Switch  Criteria=u2 > Threshold
  Unit Delay{,1..6} (7 alike) : UnitDelay  SampleTime=-1  HasFrameUpgradeWarning=on
  pdm_signal : Outport
  wires:
  [b2] -> Divide/1
  [vref] -> Divide/2
  [s1_accum] -> Unit Delay1/1
  Divide/1 -> Add/2
  [s2_accum] -> Unit Delay/1
  [a2] -> Divide1/1
  Add/1 -> Divide1/2
  Unit Delay1/1 -> Add/1
  Unit Delay/1 -> Add1/1
  Divide1/1 -> Add1/2
  [vref] -> Divide2/2
  [b1] -> Divide2/1
  Divide2/1 -> Add2/2
  [a1] -> Divide3/1
  Add2/1 -> Divide3/2
  [s1_accum] -> Unit Delay2/1
  Unit Delay2/1 -> Add3/1
  Divide3/1 -> Add3/2
  [s2_accum] -> Unit Delay3/1
  Unit Delay3/1 -> Compare To Constant/1
  Add1/1 -> Switch/1
  Add3/1 -> Switch1/1
  Switch1/1 -> [s1_accum]
  Switch/1 -> [s2_accum]
  Compare To Constant/1 -> Switch1/2, Switch/2, Switch2/2
  Switch2/1 -> [dout], pdm_signal/1
  Constant/1 -> Switch2/1
  Constant1/1 -> Switch2/3
  [s2_accum] -> Unit Delay4/1
  Unit Delay4/1 -> Add5/1
  [s1_accum] -> Unit Delay5/1
  [a2] -> Divide5/1
  [vref] -> Divide4/2
  Add4/1 -> Divide5/2
  Unit Delay5/1 -> Add4/1
  [b2] -> Divide4/1
  Add5/1 -> Switch/3
  Divide5/1 -> Add5/2
  Divide4/1 -> Add4/2
  [s1_accum] -> Unit Delay6/1
  [b1] -> Divide6/1
  Divide7/1 -> Add7/2
  Add7/1 -> Switch1/3
  [a1] -> Divide7/1
  sig_in/1 -> Add6/1, Add2/1
  Add6/1 -> Divide7/2
  Unit Delay6/1 -> Add7/1
  [vref] -> Divide6/2
  Divide6/1 -> Add6/2
  Constant2/1 -> [a2], [vref], [b1], [a1]
  Constant3/1 -> [b2]

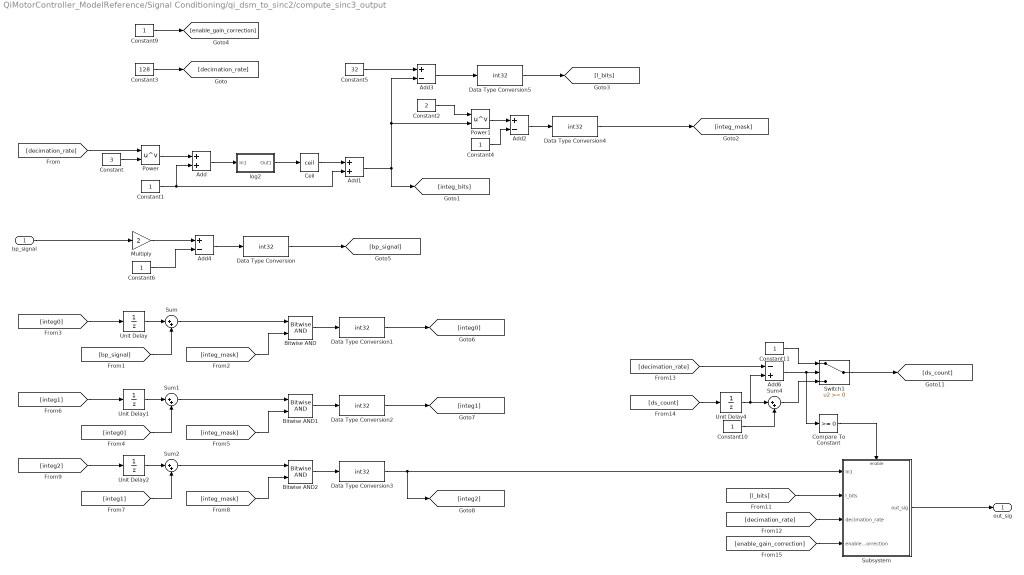
== system QiMotorController_ModelReference/Signal Conditioning/qi_dsm_to_sinc2/compute_sinc3_output ==
  bp_signal : Inport
  Add : Sum
  Add1 : Sum
  Add2 : Sum  Inputs=+-
  Add3 : Sum  Inputs=+-
  Add4 : Sum  Inputs=+-  OutDataTypeStr=int32
  Add6 : Sum  Inputs=-+  OutDataTypeStr=int32
  Bitwise AND : simulink/Logic and Bit Operations/Bitwise Operator  logicop=AND  UseBitMask=off  NumInputPorts=2  BitMask=bin2dec('11011001')  BitMaskRealWorld=Stored Integer
  Bitwise AND1 : simulink/Logic and Bit Operations/Bitwise Operator  logicop=AND  UseBitMask=off  NumInputPorts=2  BitMask=bin2dec('11011001')  BitMaskRealWorld=Stored Integer
  Bitwise AND2 : simulink/Logic and Bit Operations/Bitwise Operator  logicop=AND  UseBitMask=off  NumInputPorts=2  BitMask=bin2dec('11011001')  BitMaskRealWorld=Stored Integer
  Ceil : Rounding  Operator=ceil
  Compare To Constant : simulink/Logic and Bit Operations/Compare To Constant  relop=>=  const=0  OutDataTypeStr=boolean
  Constant : Constant  Value=3  OutDataTypeStr=single  SampleTime=-1
  Constant1 : Constant  OutDataTypeStr=single  SampleTime=-1
  Constant10 : Constant  OutDataTypeStr=int32  SampleTime=-1
  Constant11 : Constant  OutDataTypeStr=int32  SampleTime=-1
  Constant2 : Constant  Value=2  OutDataTypeStr=single  SampleTime=-1
  Constant3 : Constant  Value=128  OutDataTypeStr=single  SampleTime=-1
  Constant4 : Constant  OutDataTypeStr=single  SampleTime=-1
  Constant5 : Constant  Value=32  OutDataTypeStr=single  SampleTime=-1
  Constant6 : Constant  OutDataTypeStr=single  SampleTime=-1
  Constant9 : Constant  OutDataTypeStr=boolean  SampleTime=-1
  Data Type Conversion{,1..5} (6 alike) : DataTypeConversion  OutDataTypeStr=int32
  Multiply : Gain  Gain=2
  Power : Math  Operator=pow  SaturateOnIntegerOverflow=on
  Power1 : Math  Operator=pow  SaturateOnIntegerOverflow=on
  Subsystem : Subsystem
  Sum{,1..2,4} (4 alike) : Sum  Inputs=|++
  Switch1 : Switch
  Unit Delay : UnitDelay  SampleTime=-1  HasFrameUpgradeWarning=on
  Unit Delay1 : UnitDelay  SampleTime=-1  HasFrameUpgradeWarning=on
  Unit Delay2 : UnitDelay  SampleTime=-1  HasFrameUpgradeWarning=on
  Unit Delay4 : UnitDelay  InitialCondition=1  SampleTime=-1  HasFrameUpgradeWarning=on
  log2 : Subsystem
  out_sig : Outport
  wires:
  [decimation_rate] -> Power/1
  Constant/1 -> Power/2
  Power/1 -> Add/1
  Constant1/1 -> Add1/2, Add/2
  Constant3/1 -> [decimation_rate]
  Add/1 -> log2/1(In1)
  log2/1(Out1) -> Ceil/1
  Ceil/1 -> Add1/1
  Add1/1 -> Add3/2, Power1/2, [integ_bits]
  Constant2/1 -> Power1/1
  Power1/1 -> Add2/1
  Constant4/1 -> Add2/2
  Add2/1 -> Data Type Conversion4/1
  Constant5/1 -> Add3/1
  Add3/1 -> Data Type Conversion5/1
  bp_signal/1 -> Multiply/1
  Multiply/1 -> Add4/1
  Constant6/1 -> Add4/2
  Add4/1 -> Data Type Conversion/1
  Data Type Conversion/1 -> [bp_signal]
  Sum/1 -> Bitwise AND/1
  Unit Delay/1 -> Sum/1
  [bp_signal] -> Sum/2
  [integ_mask] -> Bitwise AND/2
  Bitwise AND/1 -> Data Type Conversion1/1
  Data Type Conversion1/1 -> [integ0]
  [integ0] -> Unit Delay/1
  Bitwise AND1/1 -> Data Type Conversion2/1
  [integ1] -> Unit Delay1/1
  [integ_mask] -> Bitwise AND1/2
  Unit Delay1/1 -> Sum1/1
  Sum1/1 -> Bitwise AND1/1
  [integ0] -> Sum1/2
  Unit Delay2/1 -> Sum2/1
  Bitwise AND2/1 -> Data Type Conversion3/1
  [integ1] -> Sum2/2
  [integ2] -> Unit Delay2/1
  Sum2/1 -> Bitwise AND2/1
  [integ_mask] -> Bitwise AND2/2
  Data Type Conversion4/1 -> [integ_mask]
  Data Type Conversion5/1 -> [l_bits]
  Constant9/1 -> [enable_gain_correction]
  Subsystem/1(out_sig) -> out_sig/1
  Sum4/1 -> Switch1/3
  Constant10/1 -> Sum4/2
  Unit Delay4/1 -> Sum4/1, Add6/2
  Constant11/1 -> Switch1/1
  Switch1/1 -> [ds_count]
  [ds_count] -> Unit Delay4/1
  [decimation_rate] -> Add6/1
  Add6/1 -> Compare To Constant/1, Switch1/2
  Compare To Constant/1 -> Subsystem/Enable
  Data Type Conversion3/1 -> [integ2], Subsystem/1(In1)
  Data Type Conversion2/1 -> [integ1]
  [l_bits] -> Subsystem/2(l_bits)
  [decimation_rate] -> Subsystem/3(decimation_rate)
  [enable_gain_correction] -> Subsystem/4(enable_gain_correction)

== system QiMotorController_ModelReference/Signal Conditioning/qi_dsm_to_sinc3/compute_dsm_output ==
  sig_in : Inport
  Add : Sum  Inputs=+-
  Add{1,3..7} (6 alike) : Sum
  Add2 : Sum  Inputs=+-
  Compare To Constant : simulink/Logic and Bit Operations/Compare To Constant  relop=>=  const=0  OutDataTypeStr=boolean
  Constant : Constant  SampleTime=-1
  Constant1 : Constant  Value=0  SampleTime=-1
  Constant2 : Constant  SampleTime=-1
  Constant3 : Constant  Value=2  SampleTime=-1
  Divide{,1..7} (8 alike) : Product  Inputs=**
  Switch : Switch  Criteria=u2 > Threshold
  Switch1 : Switch  Criteria=u2 > Threshold
  Switch2 : Switch  Criteria=u2 > Threshold
  Unit Delay{,1..6} (7 alike) : UnitDelay  SampleTime=-1  HasFrameUpgradeWarning=on
  pdm_signal : Outport
  wires:
  [b2] -> Divide/1
  [vref] -> Divide/2
  [s1_accum] -> Unit Delay1/1
  Divide/1 -> Add/2
  [s2_accum] -> Unit Delay/1
  [a2] -> Divide1/1
  Add/1 -> Divide1/2
  Unit Delay1/1 -> Add/1
  Unit Delay/1 -> Add1/1
  Divide1/1 -> Add1/2
  [vref] -> Divide2/2
  [b1] -> Divide2/1
  Divide2/1 -> Add2/2
  [a1] -> Divide3/1
  Add2/1 -> Divide3/2
  [s1_accum] -> Unit Delay2/1
  Unit Delay2/1 -> Add3/1
  Divide3/1 -> Add3/2
  [s2_accum] -> Unit Delay3/1
  Unit Delay3/1 -> Compare To Constant/1
  Add1/1 -> Switch/1
  Add3/1 -> Switch1/1
  Switch1/1 -> [s1_accum]
  Switch/1 -> [s2_accum]
  Compare To Constant/1 -> Switch1/2, Switch/2, Switch2/2
  Switch2/1 -> [dout], pdm_signal/1
  Constant/1 -> Switch2/1
  Constant1/1 -> Switch2/3
  [s2_accum] -> Unit Delay4/1
  Unit Delay4/1 -> Add5/1
  [s1_accum] -> Unit Delay5/1
  [a2] -> Divide5/1
  [vref] -> Divide4/2
  Add4/1 -> Divide5/2
  Unit Delay5/1 -> Add4/1
  [b2] -> Divide4/1
  Add5/1 -> Switch/3
  Divide5/1 -> Add5/2
  Divide4/1 -> Add4/2
  [s1_accum] -> Unit Delay6/1
  [b1] -> Divide6/1
  Divide7/1 -> Add7/2
  Add7/1 -> Switch1/3
  [a1] -> Divide7/1
  sig_in/1 -> Add6/1, Add2/1
  Add6/1 -> Divide7/2
  Unit Delay6/1 -> Add7/1
  [vref] -> Divide6/2
  Divide6/1 -> Add6/2
  Constant2/1 -> [a2], [vref], [b1], [a1]
  Constant3/1 -> [b2]

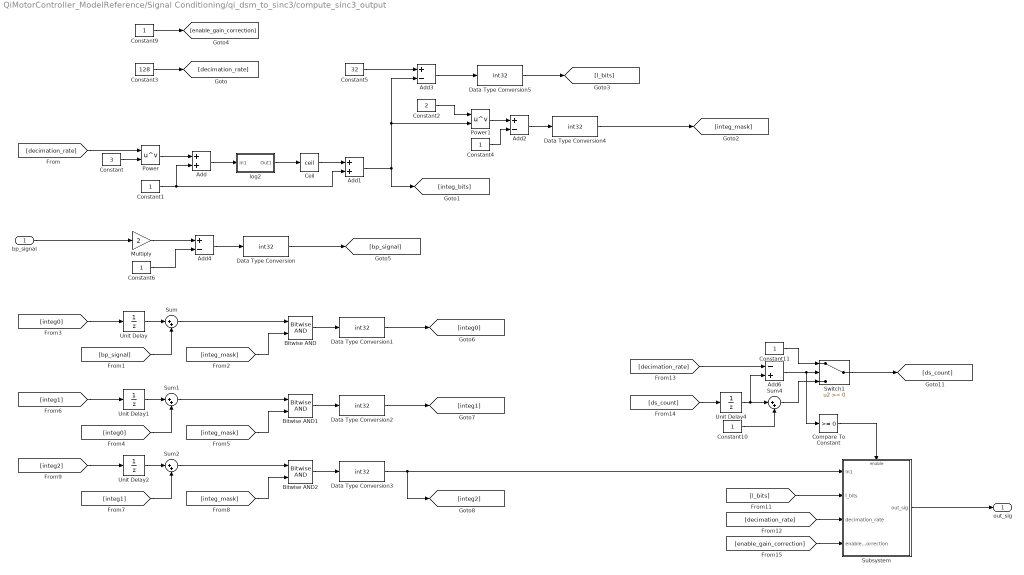
== system QiMotorController_ModelReference/Signal Conditioning/qi_dsm_to_sinc3/compute_sinc3_output ==
  bp_signal : Inport
  Add : Sum
  Add1 : Sum
  Add2 : Sum  Inputs=+-
  Add3 : Sum  Inputs=+-
  Add4 : Sum  Inputs=+-  OutDataTypeStr=int32
  Add6 : Sum  Inputs=-+  OutDataTypeStr=int32
  Bitwise AND : simulink/Logic and Bit Operations/Bitwise Operator  logicop=AND  UseBitMask=off  NumInputPorts=2  BitMask=bin2dec('11011001')  BitMaskRealWorld=Stored Integer
  Bitwise AND1 : simulink/Logic and Bit Operations/Bitwise Operator  logicop=AND  UseBitMask=off  NumInputPorts=2  BitMask=bin2dec('11011001')  BitMaskRealWorld=Stored Integer
  Bitwise AND2 : simulink/Logic and Bit Operations/Bitwise Operator  logicop=AND  UseBitMask=off  NumInputPorts=2  BitMask=bin2dec('11011001')  BitMaskRealWorld=Stored Integer
  Ceil : Rounding  Operator=ceil
  Compare To Constant : simulink/Logic and Bit Operations/Compare To Constant  relop=>=  const=0  OutDataTypeStr=boolean
  Constant : Constant  Value=3  OutDataTypeStr=single  SampleTime=-1
  Constant1 : Constant  OutDataTypeStr=single  SampleTime=-1
  Constant10 : Constant  OutDataTypeStr=int32  SampleTime=-1
  Constant11 : Constant  OutDataTypeStr=int32  SampleTime=-1
  Constant2 : Constant  Value=2  OutDataTypeStr=single  SampleTime=-1
  Constant3 : Constant  Value=128  OutDataTypeStr=single  SampleTime=-1
  Constant4 : Constant  OutDataTypeStr=single  SampleTime=-1
  Constant5 : Constant  Value=32  OutDataTypeStr=single  SampleTime=-1
  Constant6 : Constant  OutDataTypeStr=single  SampleTime=-1
  Constant9 : Constant  OutDataTypeStr=boolean  SampleTime=-1
  Data Type Conversion{,1..5} (6 alike) : DataTypeConversion  OutDataTypeStr=int32
  Multiply : Gain  Gain=2
  Power : Math  Operator=pow  SaturateOnIntegerOverflow=on
  Power1 : Math  Operator=pow  SaturateOnIntegerOverflow=on
  Subsystem : Subsystem
  Sum{,1..2,4} (4 alike) : Sum  Inputs=|++
  Switch1 : Switch
  Unit Delay : UnitDelay  SampleTime=-1  HasFrameUpgradeWarning=on
  Unit Delay1 : UnitDelay  SampleTime=-1  HasFrameUpgradeWarning=on
  Unit Delay2 : UnitDelay  SampleTime=-1  HasFrameUpgradeWarning=on
  Unit Delay4 : UnitDelay  InitialCondition=1  SampleTime=-1  HasFrameUpgradeWarning=on
  log2 : Subsystem
  out_sig : Outport
  wires:
  [decimation_rate] -> Power/1
  Constant/1 -> Power/2
  Power/1 -> Add/1
  Constant1/1 -> Add1/2, Add/2
  Constant3/1 -> [decimation_rate]
  Add/1 -> log2/1(In1)
  log2/1(Out1) -> Ceil/1
  Ceil/1 -> Add1/1
  Add1/1 -> Add3/2, Power1/2, [integ_bits]
  Constant2/1 -> Power1/1
  Power1/1 -> Add2/1
  Constant4/1 -> Add2/2
  Add2/1 -> Data Type Conversion4/1
  Constant5/1 -> Add3/1
  Add3/1 -> Data Type Conversion5/1
  bp_signal/1 -> Multiply/1
  Multiply/1 -> Add4/1
  Constant6/1 -> Add4/2
  Add4/1 -> Data Type Conversion/1
  Data Type Conversion/1 -> [bp_signal]
  Sum/1 -> Bitwise AND/1
  Unit Delay/1 -> Sum/1
  [bp_signal] -> Sum/2
  [integ_mask] -> Bitwise AND/2
  Bitwise AND/1 -> Data Type Conversion1/1
  Data Type Conversion1/1 -> [integ0]
  [integ0] -> Unit Delay/1
  Bitwise AND1/1 -> Data Type Conversion2/1
  [integ1] -> Unit Delay1/1
  [integ_mask] -> Bitwise AND1/2
  Unit Delay1/1 -> Sum1/1
  Sum1/1 -> Bitwise AND1/1
  [integ0] -> Sum1/2
  Unit Delay2/1 -> Sum2/1
  Bitwise AND2/1 -> Data Type Conversion3/1
  [integ1] -> Sum2/2
  [integ2] -> Unit Delay2/1
  Sum2/1 -> Bitwise AND2/1
  [integ_mask] -> Bitwise AND2/2
  Data Type Conversion4/1 -> [integ_mask]
  Data Type Conversion5/1 -> [l_bits]
  Constant9/1 -> [enable_gain_correction]
  Subsystem/1(out_sig) -> out_sig/1
  Sum4/1 -> Switch1/3
  Constant10/1 -> Sum4/2
  Unit Delay4/1 -> Sum4/1, Add6/2
  Constant11/1 -> Switch1/1
  Switch1/1 -> [ds_count]
  [ds_count] -> Unit Delay4/1
  [decimation_rate] -> Add6/1
  Add6/1 -> Compare To Constant/1, Switch1/2
  Compare To Constant/1 -> Subsystem/Enable
  Data Type Conversion3/1 -> [integ2], Subsystem/1(In1)
  Data Type Conversion2/1 -> [integ1]
  [l_bits] -> Subsystem/2(l_bits)
  [decimation_rate] -> Subsystem/3(decimation_rate)
  [enable_gain_correction] -> Subsystem/4(enable_gain_correction)

== system QiMotorController_ModelReference/Signal Conditioning/qi_dsm_to_sinc4/compute_dsm_output ==
  sig_in : Inport
  Add : Sum  Inputs=+-
  Add{1,3..7} (6 alike) : Sum
  Add2 : Sum  Inputs=+-
  Compare To Constant : simulink/Logic and Bit Operations/Compare To Constant  relop=>=  const=0  OutDataTypeStr=boolean
  Constant : Constant  SampleTime=-1
  Constant1 : Constant  Value=0  SampleTime=-1
  Constant2 : Constant  SampleTime=-1
  Constant3 : Constant  Value=2  SampleTime=-1
  Divide{,1..7} (8 alike) : Product  Inputs=**
  Switch : Switch  Criteria=u2 > Threshold
  Switch1 : Switch  Criteria=u2 > Threshold
  Switch2 : Switch  Criteria=u2 > Threshold
  Unit Delay{,1..6} (7 alike) : UnitDelay  SampleTime=-1  HasFrameUpgradeWarning=on
  pdm_signal : Outport
  wires:
  [b2] -> Divide/1
  [vref] -> Divide/2
  [s1_accum] -> Unit Delay1/1
  Divide/1 -> Add/2
  [s2_accum] -> Unit Delay/1
  [a2] -> Divide1/1
  Add/1 -> Divide1/2
  Unit Delay1/1 -> Add/1
  Unit Delay/1 -> Add1/1
  Divide1/1 -> Add1/2
  [vref] -> Divide2/2
  [b1] -> Divide2/1
  Divide2/1 -> Add2/2
  [a1] -> Divide3/1
  Add2/1 -> Divide3/2
  [s1_accum] -> Unit Delay2/1
  Unit Delay2/1 -> Add3/1
  Divide3/1 -> Add3/2
  [s2_accum] -> Unit Delay3/1
  Unit Delay3/1 -> Compare To Constant/1
  Add1/1 -> Switch/1
  Add3/1 -> Switch1/1
  Switch1/1 -> [s1_accum]
  Switch/1 -> [s2_accum]
  Compare To Constant/1 -> Switch1/2, Switch/2, Switch2/2
  Switch2/1 -> [dout], pdm_signal/1
  Constant/1 -> Switch2/1
  Constant1/1 -> Switch2/3
  [s2_accum] -> Unit Delay4/1
  Unit Delay4/1 -> Add5/1
  [s1_accum] -> Unit Delay5/1
  [a2] -> Divide5/1
  [vref] -> Divide4/2
  Add4/1 -> Divide5/2
  Unit Delay5/1 -> Add4/1
  [b2] -> Divide4/1
  Add5/1 -> Switch/3
  Divide5/1 -> Add5/2
  Divide4/1 -> Add4/2
  [s1_accum] -> Unit Delay6/1
  [b1] -> Divide6/1
  Divide7/1 -> Add7/2
  Add7/1 -> Switch1/3
  [a1] -> Divide7/1
  sig_in/1 -> Add6/1, Add2/1
  Add6/1 -> Divide7/2
  Unit Delay6/1 -> Add7/1
  [vref] -> Divide6/2
  Divide6/1 -> Add6/2
  Constant2/1 -> [a2], [vref], [b1], [a1]
  Constant3/1 -> [b2]
